simulink model "sasprojectsimulink"  (R2018b)
settings: Solver=VariableStepAuto  StartTime=0.0  StopTime=10  RelTol=1e-3  EnableMultiTasking=on
values from neighbouring files (symbols this model uses):
  A1 = 0.00292    [sasproj.m]
  A2 = 0.000633    [sasproj.m]
  F = zeros(m,n)    [sasproj.m]
  mass = 12.3    [sasproj.m]
  p0 = 2.0684*(10^7)    (= 20684000)    [sasproj.m]
  sigma = [-15:1:15]    [sasproj.m]
  v = [180:5:330]    [sasproj.m]
  x = h*(sind(sigma))    [sasproj.m]
undefined symbols (not defined in the file or in its folder): sigbuilder_block
libraries: simulink x2
settings Model: Creator=student  LastModifiedBy=enock
settings DataIOCC: LimitDataPoints=on
settings OptimizationCC: LifeSpan=inf
settings DebuggingCC: AllowSymbolicDim=off  SFUnexpectedBacktrackingDiag=warning  SFNoUnconditionalDefaultTransitionDiag=warning  SFExecutionAtInitializationDiag=none
settings ModelReferenceCC: PropagateSignalLabelsOutOfModel=off
settings SFSimCC: SimUseLocalCustomCode=off
settings RTWCC: RTWUseLocalCustomCode=off
settings CodeAppCC: StateflowObjectComments=on
settings GRTTargetCC: TargetLangStandard=C89/C90 (ANSI)
settings ConfigComp: CovMetricSettings=dw  CovHtmlReporting=on  CovSaveCumulativeToWorkspaceVar=on  CovSaveSingleToWorkspaceVar=on  CovExternalEMLEnable=off

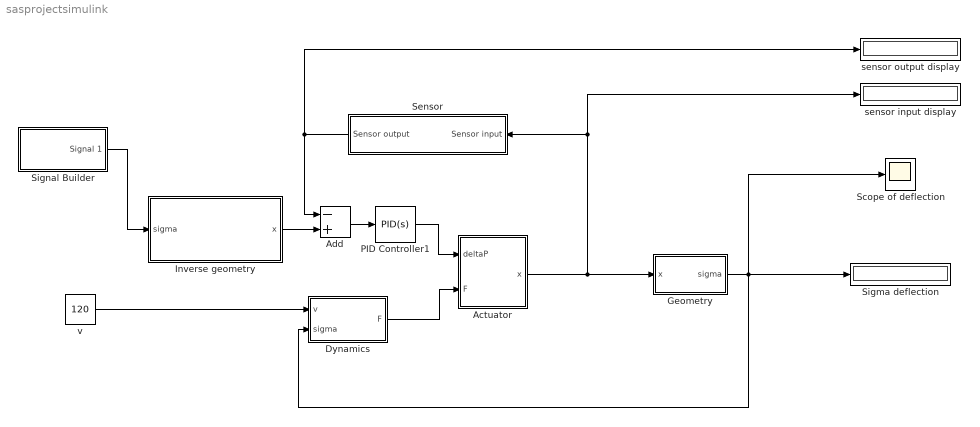
== system sasprojectsimulink ==
  Actuator : Subsystem
  Add : Sum  Inputs=-+
  "Dynamics " : Subsystem
  "Geometry " : Subsystem
  "Inverse geometry " : Subsystem
  PID Controller1 : simulink/Continuous/PID Controller  Controller=PID  Form=Parallel  TimeDomain=Continuous-time  SampleTime=-1  IntegratorMethod=Forward Euler  FilterMethod=Forward Euler  ControllerParametersSource=internal  P=-66372629040.9353  I=-13268822233317  D=-81524652.0709093  UseFilter=on  N=23290.1963199526  TunerSelectOption=Transfer Function Based (PID Tuner App)  InitialConditionSource=internal  InitialConditionForIntegrator=0  InitialConditionForFilter=0  DifferentiatorICPrevScaledInput=0  ExternalReset=none  TrackingMode=off  Kt=1  LimitOutput=off  UpperSaturationLimit=inf  LowerSaturationLimit=-inf  LinearizeAsGain=on  AntiWindupMode=none  Kb=1  POutMin=[]  POutMax=[]  IOutMin=[]  IOutMax=[]  DOutMin=[]  DOutMax=[]  NOutMin=[]  NOutMax=[]  SumOutMin=[]  SumOutMax=[]  SaturationOutMin=[]  SaturationOutMax=[]  PParamMin=[]  PParamMax=[]  IParamMin=[]  IParamMax=[]  DParamMin=[]  DParamMax=[]  NParamMin=[]  NParamMax=[]  KbParamMin=[]  KbParamMax=[]  KtParamMin=[]  KtParamMax=[]  KbOutMin=[]  KbOutMax=[]  KtOutMin=[]  KtOutMax=[]  IntegratorOutMin=[]  IntegratorOutMax=[]  FilterOutMin=[]  FilterOutMax=[]  SumI1OutMin=[]  SumI1OutMax=[]  SumI2OutMin=[]  SumI2OutMax=[]  SumI3OutMin=[]  SumI3OutMax=[]  SumI4OutMin=[]  SumI4OutMax=[]  SumDOutMin=[]  SumDOutMax=[]  DifferentiatorOutMin=[]  DifferentiatorOutMax=[]  FilterDiffOutCoefMin=[]  FilterDiffOutCoefMax=[]  ReciprocalOutMin=[]  ReciprocalOutMax=[]  SumDenOutMin=[]  SumDenOutMax=[]  SumNumOutMin=[]  SumNumOutMax=[]  DivideOutMin=[]  DivideOutMax=[]  IntegratorContinuousStateAttributes=''  IntegratorStateMustResolveToSignalObject=off  IntegratorRTWStateStorageClass=Auto  FilterContinuousStateAttributes=''  FilterStateMustResolveToSignalObject=off  FilterRTWStateStorageClass=Auto  ParallelPVariant=InternalParameters  IdealPVariant=Disabled  IVariant=InternalParameters  DVariant=InternalParameters  IntegratorVariant=Continuous  SatVariant=Disabled  AWVariant=Passthrough  PCopyVariant=Disabled  TRVariant=Disabled  FdbkBlocksVariant=Forward  IdealPFdbkVariant=Disabled  SatFdbkVariant=Disabled  DerivativeFilterVariant=ContFilter  NVariant=InternalParameters  NCopyVariant=Disabled  FilterICVariant=InternalICsFilter  IntegratorICVariant=InternalICs  ExternalResetVariant=Disabled  TRSumVariant=Passthrough  SumFdbkVariant=Disabled  SumVariant=Sum_PID
  Scope of deflection : Scope
  "Sensor " : Subsystem
  Sigma deflection : Display
  Signal Builder : Subsystem  Tag=STV Subsys  LoadFcn=sigbuilder_block('load');  StartFcn=sigbuilder_block('start');  StopFcn=sigbuilder_block('stop');  ClipboardFcn=sigbuilder_block('clipboard');  mask(Sigbuilder block){tuvar=[0:10]}
      mask help: Simulink:masks:SigbuilderBlock_MD
      mask init:
      | if ~strcmp(get_param(bdroot(gcbh),'SimulationStatus'),'stopped') tuvar = sigbuilder_block('maskInit'); end
      settings: CopyFcn=sigbuilder_block('copy');  DeleteFcn=sigbuilder_block('delete');  ModelCloseFcn=sigbuilder_block('modelClose');  PreSaveFcn=sigbuilder_block('preSave');  PauseFcn=sigbuilder_block('pause');  ContinueFcn=sigbuilder_block('continue');  NameChangeFcn=sigbuilder_block('namechange');  OpenFcn=sigbuilder_block('open',[-862.8 -6 550.8 244.2 ]);  CloseFcn=sigbuilder_block('close');
      mask Display: plot(0, 0, 100, 100,[2, 2, 32, 32, 2], [68, 8, 8, 68, 68],[32, 2], [38, 38], [32, 19, 2],[53, 60, 44], [32, 17, 17, 2],[16, 16, 31, 31]);txt = getActiveGroup(gcbh);text(2, 100, txt,'verticalAlignment', 'top');
  "sensor input display  " : Display
  "sensor output display " : Display
  v : Constant  Value=120
  wires:
  "Geometry "/1(sigma) -> Scope of deflection/1, Sigma deflection/1, "Dynamics "/2("sigma ")
  "Dynamics "/1(F) -> Actuator/2(F)
  "Inverse geometry "/1(x) -> Add/2
  v/1 -> "Dynamics "/1(v)
  "Sensor "/1(Sensor output) -> Add/1, "sensor output display "/1
  Actuator/1(x) -> "sensor input display  "/1, "Sensor "/1(Sensor input), "Geometry "/1(x)
  Add/1 -> PID Controller1/1
  PID Controller1/1 -> Actuator/1("deltaP ")
  Signal Builder/1(Signal 1) -> "Inverse geometry "/1(sigma)

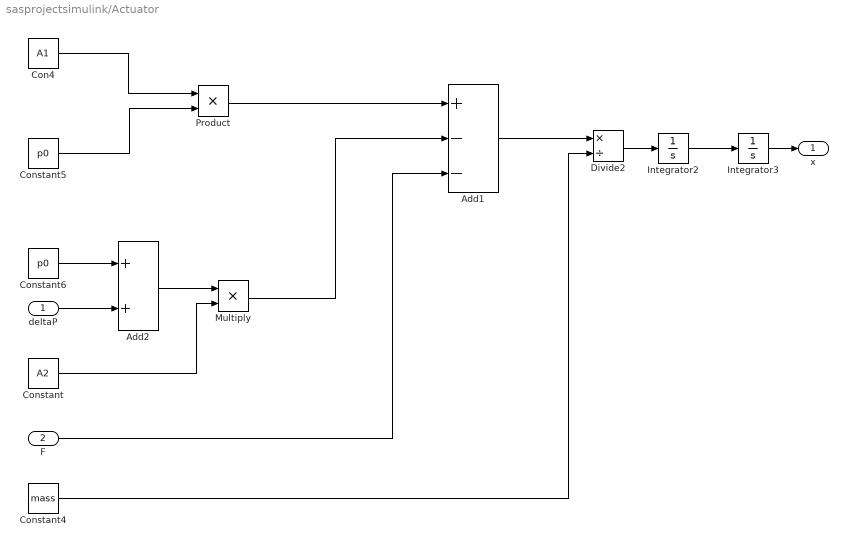
== system sasprojectsimulink/Actuator ==
  "deltaP " : Inport
  F : Inport  Port=2
  Add1 : Sum  Inputs=+--
  Add2 : Sum
  Con4 : Constant  Value=A1
  Constant : Constant  Value=A2
  Constant4 : Constant  Value=mass
  Constant5 : Constant  Value=p0
  Constant6 : Constant  Value=p0  LockScale=on
  Divide2 : Product  Inputs=*/
  Integrator2 : Integrator
  Integrator3 : Integrator
  Multiply : Product
  Product : Product
  x : Outport
  wires:
  F/1 -> Add1/3
  Product/1 -> Add1/1
  Multiply/1 -> Add1/2
  Constant/1 -> Multiply/2
  Con4/1 -> Product/1
  Constant4/1 -> Divide2/2
  Integrator3/1 -> x/1
  Constant6/1 -> Add2/1
  Add2/1 -> Multiply/1
  "deltaP "/1 -> Add2/2
  Constant5/1 -> Product/2
  Integrator2/1 -> Integrator3/1
  Divide2/1 -> Integrator2/1
  Add1/1 -> Divide2/1

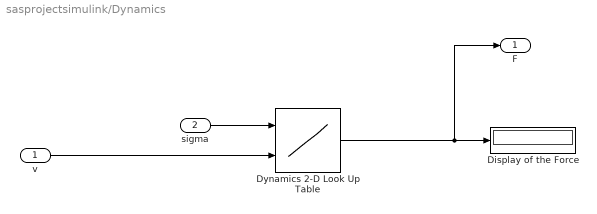
== system sasprojectsimulink/Dynamics  ==
  v : Inport
  "sigma " : Inport  Port=2
  "Display of the Force " : Display
  Dynamics 2-D Look Up Table : Lookup_n-D  BreakpointsForDimension1=sigma  BreakpointsForDimension2=v  Table=F  InternalRulePriority=Speed  RndMeth=Simplest  InputSameDT=on
  F : Outport
  wires:
  v/1 -> Dynamics 2-D Look Up Table/2
  Dynamics 2-D Look Up Table/1 -> F/1, "Display of the Force "/1
  "sigma "/1 -> Dynamics 2-D Look Up Table/1

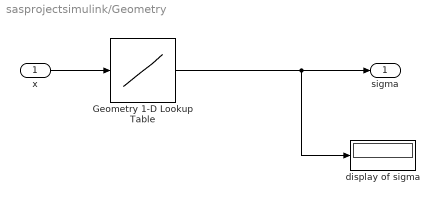
== system sasprojectsimulink/Geometry  ==
  x : Inport
  Geometry 1-D Lookup Table : Lookup_n-D  NumberOfTableDimensions=1  BreakpointsForDimension1=x  Table=sigma  InternalRulePriority=Speed  RndMeth=Simplest  InputSameDT=on
  display of sigma : Display
  sigma : Outport
  wires:
  x/1 -> Geometry 1-D Lookup Table/1
  Geometry 1-D Lookup Table/1 -> display of sigma/1, sigma/1

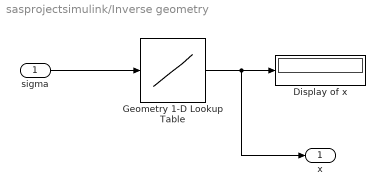
== system sasprojectsimulink/Inverse geometry  ==
  sigma : Inport
  "Display of x " : Display
  Geometry 1-D Lookup Table : Lookup_n-D  NumberOfTableDimensions=1  BreakpointsForDimension1=sigma  Table=x  InternalRulePriority=Speed  RndMeth=Simplest  InputSameDT=on
  x : Outport
  wires:
  sigma/1 -> Geometry 1-D Lookup Table/1
  Geometry 1-D Lookup Table/1 -> x/1, "Display of x "/1

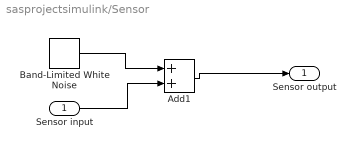
== system sasprojectsimulink/Sensor  ==
  Sensor input : Inport
  Add1 : Sum
  Band-Limited White Noise : simulink/Sources/Band-Limited White Noise  Cov=0.0000000002  Ts=0.0001  seed=1
  Sensor output : Outport
  wires:
  Sensor input/1 -> Add1/2
  Add1/1 -> Sensor output/1
  Band-Limited White Noise/1 -> Add1/1

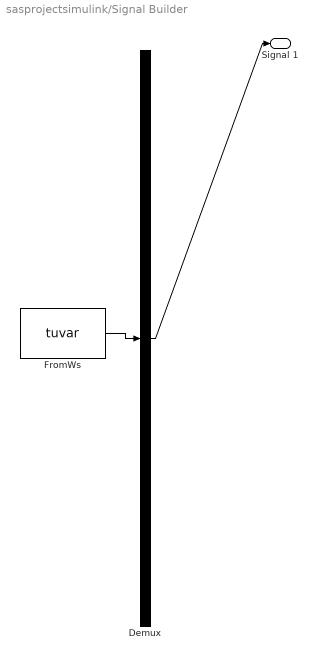
== system sasprojectsimulink/Signal Builder ==
  Demux : Demux  Tag=STV Demux  Outputs=1
  FromWs : FromWorkspace  Tag=STV FromWs  VariableName=tuvar  SampleTime=0
      SigBuilderData=|
      | common.afterFinalStr = 'Extrapolate'
      | common.sampleTime = 0
      | dataSet.timeRange = [0 10]
      | dataSet.name = 'Group 1'
      | sbobj.Groups.Name = 'Group 1'
      | sbobj.Groups.Signals.Name = 'Signal 1'
      | sbobj.Groups.Signals.XData = [0 4 4 6 6 10]
      | sbobj.Groups.Signals.YData = [0 -10.6 1.2 10.75 4.6 0]
  Signal 1 : Outport  Tag=STV Outport
  wires:
  FromWs/1 -> Demux/1
  Demux/1 -> Signal 1/1
